simulink model "tyre_model_v3"  (R2024b)
settings: Solver=FixedStepAuto  StartTime=0.0  StopTime=10.0  FixedStep=Ts  MaxStep=0.001  RelTol=1e-3
values from neighbouring files (symbols this model uses):
  Re = 0.235    [main_data_vehicle.m]    (also in xopt_launch.mat)
  v0 = 0    [main_data_vehicle.m]    (also in xopt_launch.mat)
libraries: vehdynlibtire x1
settings Model: Creator=marti  LastModifiedBy=marti

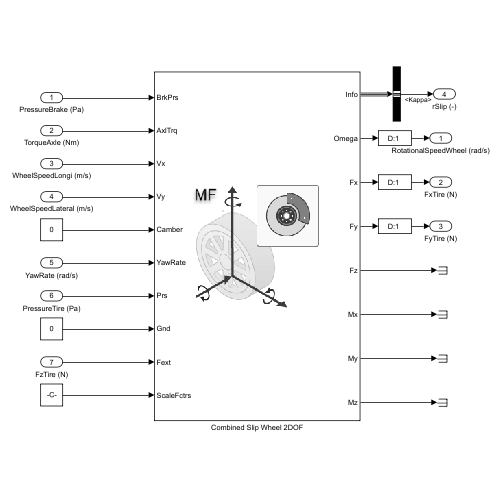
[thumbnail: Simulink's stored preview of the top-level diagram]
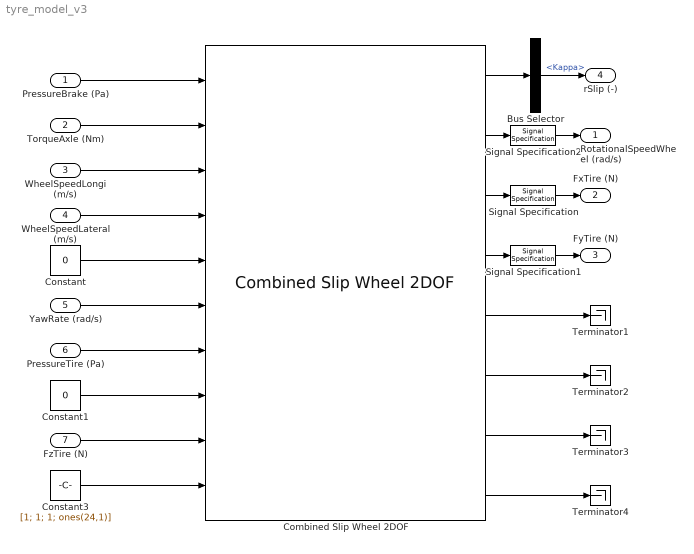
== system tyre_model_v3 ==
  PressureBrake (Pa) : Inport
  TorqueAxle (Nm) : Inport  Port=2
  WheelSpeedLongi (m/s) : Inport  Port=3
  WheelSpeedLateral (m/s) : Inport  Port=4
  YawRate (rad/s) : Inport  Port=5
  PressureTire (Pa) : Inport  Port=6
  FzTire (N) : Inport  Port=7
  Bus Selector : BusSelector  OutputSignals=Kappa
  Combined Slip Wheel 2DOF : vehdynlibtire/Combined Slip Wheel 2DOF  tireType=External file  tireParamSet=C:\Users\marti\Documents\EPSA\GIT\R-D\Commande bimoteur\2025 - Martin\Post stage\Optimisation LS\Car model\GoodyearR13Updated.tir  vertType=Magic Formula  plySteer=off  turnslip=off  BrakeType=Disc  mu_static=.3  mu_kinetic=.2  drum_abore=0.0508  drum_a=0.123  drum_c=0.212  drum_r=0.15  drum_theta1=0  drum_theta2=126  disk_abore=.05  Rm=.177  num_pads=2  brake_p_bpt=[1 11.4736842105263 21.9473684210526 32.4210526315789 42.8947368421053 53.3684210526316 63.8421052631579 74.3157894736842 84.7894736842105 95.2631578947368 105.736842105263 116.210526315789 126.684210526316 137.157894736842 147.631578947368 158.105263157895 168.578947368421 179.052631578947 189.526315789474 200]  brake_n_bpt=[0 52.6315789473684 105.263157894737 157.894736842105 210.526315789474 263.157894736842 315.789473684211 368.421052631579 421.052631578947 473.684210526316 526.315789473684 578.947368421053 631.578947368421 684.210526315789 736.842105263158 789.473684210526 842.105263157895 894.736842105263 947.368421052632 1000]  f_brake_t=[43.4900602404453 42.5056030554862 41.5350898940194 40.5780454442085 39.6340111501808 38.7025443887544 37.7832176914519 36.8756180088306 35.9793460143796 35.0940154454303 34.2192524787115 33.3546951383474 32.4999927342521 31.6548053290159 30.8188032315107 29.991666515561 29.1730845621415 28.362755623661 27.5603864089927 26.765691687993;498.991217495636 487.695866636631 476.560505099801 465.579679307235 454.748127933653 444.060772460445 433.51270824929 423.099196101319 412.81565427025 402.657650900201 392.620896861006 382.701238955775 372.894653477208 363.197240090814 353.605216024701 344.114910546964 334.722759712992 325.425301366216 316.219170376863 307.10109410434;954.492374750826 932.886130217776 911.585920305583 890.581313170261 869.862244717126 849.419000532136 829.242198807128 809.322774193808 789.651962526121 770.221286354971 751.0225412433 732.047782773203 713.289314220164 694.739674852612 676.391628817892 658.238154578366 640.272434863842 622.48784710877 604.877954344734 587.436496520688;1409.99353200602 1378.07639379892 1346.61133551136 1315.58294703329 1284.9763615006 1254.77722860383 1224.97168936497 1195.5463522863 1166.48827078199 1137.78492180974 1109.42418562559 1081.39432659063 1053.68397496312 1026.28210961441 999.178041611083 972.361398609768 945.822110014692 919.550392851325 893.536738312604 867.771898937035;1865.49468926121 1823.26665738007 1781.63675071715 1740.58458089631 1700.09047828407 1660.13545667552 1620.7011799228 1581.76993037878 1543.32457903786 1505.34855726451 1467.82583000789 1430.74087040806 1394.07863570608 1357.82454437621 1321.96445440427 1286.48464264117 1251.37178516554 1216.61293859388 1182.19552228048 1148.10730135338;2320.9958465164 2268.45692096121 2216.66216592293 2165.58621475934 2115.20459506754 2065.49368474721 2016.43067048064 1967.99350847127 1920.16088729373 1872.91219271928 1826.22747439018 1780.08741422549 1734.47329644903 1689.36697913801 1644.75086719747 1600.60788667257 1556.92146031639 1513.67548433643 1470.85430624835 1428.44270376973;2776.49700377159 2713.64718454235 2651.68758112871 2590.58784862237 2530.31871185102 2470.8519128189 2412.16016103848 2354.21708656376 2296.9971955496 2240.47582817405 2184.62911877248 2129.43395804292 2074.86795719199 2020.9094138998 1967.53727999066 1914.73113070398 1862.47113546724 1810.73803007899 1759.51309021622 1708.77810618608;3231.99816102678 3158.8374481235 3086.71299633449 3015.58948248539 2945.43282863449 2876.21014089059 2807.88965159632 2740.44066465625 2673.83350380547 2608.03946362882 2543.03076315477 2478.78050186034 2415.26261793494 2352.4518486616 2290.32369278385 2228.85437473538 2168.02081061809 2107.80057582154 2048.17187418409 1989.11350860242;3687.49931828197 3604.02771170464 3521.73841154027 3440.59111634842 3360.54694541796 3281.56836896228 3203.61914215416 3126.66424274874 3050.66981206134 2975.60309908359 2901.43240753707 2828.12704567777 2755.6572786779 2683.9942834234 2613.11010557704 2542.97761876678 2473.57048576894 2404.8631215641 2336.83065815196 2269.44891101877;4143.00047553716 4049.21797528579 3956.76382674606 3865.59275021144 3775.66106220143 3686.92659703397 3599.34863271199 3512.88782084123 3427.50612031721 3343.16673453836 3259.83405191936 3177.4735894952 3096.05193942085 3015.5367181852 2935.89651837023 2857.10086279818 2779.12016091979 2701.92566730665 2625.48944211983 2549.78431343512;4598.50163279235 4494.40823886693 4391.78924195184 4290.59438407447 4190.77517898491 4092.28482510566 3995.07812326983 3899.11139893372 3804.34242857308 3710.73036999313 3618.23569630166 3526.82013331263 3436.44660016381 3347.079152947 3258.68293116342 3171.22410682959 3084.66983607064 2998.98821304921 2914.1482260877 2830.11971585147;5054.00279004754 4939.59850244808 4826.81465715762 4715.59601793749 4605.88929576838 4497.64305317735 4390.80761382767 4285.3349770262 4181.17873682896 4078.2940054479 3976.63734068395 3876.16667713006 3776.84126090677 3678.62158770879 3581.46934395661 3485.34735086099 ...(+2764 chars)]  NOMPRES=100000  PRESMAX=413685.6  PRESMIN=0  FNOMIN=800  FZMAX=1600  FZMIN=228.6  VXLOW=1  KPUMAX=1  KPUMIN=-1  ALPMAX=0.2094  ALPMIN=-0.2094  CAMMAX=0.1047  CAMMIN=-0.1047  LONGVL=10  FxRelFreqLwrLim=200*pi  FyRelFreqLwrLim=200*pi  MyRelFreqLwrLim=100*pi  omegao=v0/Re  UNLOADED_RADIUS=0.259  WIDTH=0.177  RIM_RADIUS=0.165  ASPECT_RATIO=53  MASS=7  IYY=J  br=1e-3  GRAVITY=-9.81  zo=0  zdoto=0  BREFF=3.811  DREFF=0.4088  FREFF=0.03564  Q_RE0=1.003  Q_V1=0.000864  Q_V2=0.025807  Q_FZ1=0  Q_FZ2=51.51  Q_FZ3=0  Q_FCX=0  Q_FCY=0  Q_FCY2=0  PFZ1=1  VERTICAL_STIFFNESS=86000  VERTICAL_DAMPING=3885  BOTTOM_OFFST=0.01  BOTTOM_STIFF=2000000  Q_CAM1=0  Q_CAM2=0  Q_CAM3=0  Q_FYS1=0  Q_FYS2=0  Q_FYS3=0  LONGITUDINAL_STIFFNESS=505632.6  LATERAL_STIFFNESS=219162.7  PCFX1=-0.12193  PCFX2=0  PCFX3=0  PCFY1=-0.17034  PCFY2=0  PCFY3=0  Q_RA1=0.602  Q_RA2=1.024  Q_RB1=1.1137  Q_RB2=-0.09748  PCX1=1.532  PDX1=2.0217  PDX2=-4.4519e-13  PDX3=4.9582e-12  PEX1=-0.53967  PEX2=0.033899  PEX3=0.6  PEX4=-0.9  PKX1=31.5328  PKX2=18.3602  PKX3=-0.83512  PHX1=-0.0018797  PHX2=-0.0030287  PVX1=0.021199  PVX2=-0.016041  PPX1=-7.3979  PPX2=-21.4276  PPX3=-3.4788  PPX4=-9.3616  RBX1=7.2469  RBX2=7.3187  RBX3=293.6691  RCX1=1.2  REX1=-1.4799  REX2=1  RHX1=0.010551  QSX1=-0.0045595  QSX2=1.0969  QSX3=0.083179  QSX4=0.27961  QSX5=0  QSX6=0  QSX7=0.26836  QSX8=0  QSX9=0  QSX10=0  QSX11=0  QSX12=0  QSX13=0  QSX14=0  PPMX1=0.31908  PCY1=2.2759  PDY1=2.3528  PDY2=-0.29552  PDY3=-0.45204  PEY1=1.4836  PEY2=0.30607  PEY3=0.093739  PEY4=0.044259  PEY5=9.9714  PKY1=-41.0748  PKY2=1.3976  PKY3=0.85032  PKY4=1.5914  PKY5=4.2457  PKY6=-5.0674  PKY7=-2.9549  PHY1=0.00079017  PHY2=0.0075541  PVY1=0.093488  PVY2=-0.01165  PVY3=1.6546  PVY4=2.0195  PPY1=1.0167  PPY2=1.8408  PPY3=-0.19906  PPY4=-0.04479  PPY5=0.62429  RBY1=20.0011  RBY2=11.7932  RBY3=0.060495  RBY4=89.998  RCY1=0.82412  REY1=-0.77168  REY2=-1  RHY1=0.021878  RHY2=0.053297  RVY1=0  RVY2=0  RVY3=0  RVY4=0  RVY5=0  RVY6=0  QSY1=0  QSY2=0  QSY3=0  QSY4=0  QSY5=0  QSY6=0  QSY7=0.85  QSY8=-0.4  QBZ1=0.10359  QBZ2=-0.0055847  QBZ3=-0.012184  QBZ4=0.49461  QBZ5=0.49461  QBZ6=0  QBZ9=20.1937  QBZ10=0.59001  QCZ1=7.1199  QDZ1=0.077371  QDZ2=-0.012902  QDZ3=1.9167  QDZ4=-10.3858  QDZ6=0.0063923  QDZ7=-0.041559  QDZ8=-1.9454  QDZ9=3.3525  QDZ10=3.2841  QDZ11=-2.483  QEZ1=-0.012366  QEZ2=-0.025481  QEZ3=-0.013833  QEZ4=-0.0049145  QEZ5=-0.0020112  QHZ1=-0.29861  QHZ2=-0.083794  QHZ3=1.7598  QHZ4=0.47757  PPZ1=-4.0641  PPZ2=-1.804  SSZ1=-0.024675  SSZ2=-0.06007  SSZ3=0  SSZ4=0  PDXP1=0  PDXP2=0  PDXP3=0  PKYP1=0  PDYP1=0  PDYP2=0  PDYP3=0  PDYP4=0  PHYP1=0  PHYP2=0  PHYP3=0  PHYP4=0  PECP1=0  PECP2=0  QDTP1=0  QCRP1=0  QCRP2=0  QBRP1=0  QDRP1=0  QDRP2=0  aMode=2
  Constant : Constant  Value=0
  Constant1 : Constant  Value=0
  Constant3 : Constant  Value=[1; 1; 1; ones(24,1)]
  Signal Specification : SignalSpecification  Dimensions=1
  Signal Specification1 : SignalSpecification  Dimensions=1
  Signal Specification2 : SignalSpecification  Dimensions=1
  Terminator{1..4} (4 alike) : Terminator
  RotationalSpeedWheel (rad/s) : Outport
  FxTire (N) : Outport  Port=2
  FyTire (N) : Outport  Port=3
  rSlip (-) : Outport  Port=4
  wires:
  PressureBrake (Pa)/1 -> Combined Slip Wheel 2DOF/1
  TorqueAxle (Nm)/1 -> Combined Slip Wheel 2DOF/2
  WheelSpeedLongi (m/s)/1 -> Combined Slip Wheel 2DOF/3
  WheelSpeedLateral (m/s)/1 -> Combined Slip Wheel 2DOF/4
  Constant/1 -> Combined Slip Wheel 2DOF/5
  YawRate (rad/s)/1 -> Combined Slip Wheel 2DOF/6
  PressureTire (Pa)/1 -> Combined Slip Wheel 2DOF/7
  Constant1/1 -> Combined Slip Wheel 2DOF/8
  FzTire (N)/1 -> Combined Slip Wheel 2DOF/9
  Constant3/1 -> Combined Slip Wheel 2DOF/10
  Combined Slip Wheel 2DOF/1 -> Bus Selector/1
  Combined Slip Wheel 2DOF/2 -> Signal Specification2/1
  Combined Slip Wheel 2DOF/3 -> Signal Specification/1
  Combined Slip Wheel 2DOF/4 -> Signal Specification1/1
  Combined Slip Wheel 2DOF/5 -> Terminator1/1
  Combined Slip Wheel 2DOF/6 -> Terminator2/1
  Combined Slip Wheel 2DOF/7 -> Terminator3/1
  Combined Slip Wheel 2DOF/8 -> Terminator4/1
  Signal Specification/1 -> FxTire (N)/1
  Signal Specification1/1 -> FyTire (N)/1
  Signal Specification2/1 -> RotationalSpeedWheel (rad/s)/1
  Bus Selector/1 -> rSlip (-)/1  "<Kappa>"
